simulink model "fmcw_rangemodel.slx"  (R2024b)
settings: Solver=FixedStepDiscrete  StartTime=0.0  StopTime=1.28e-3  FixedStep=5e-9  RelTol=1e-3
undefined symbols (not defined in the file or in its folder): physconst
libraries: phasedenvlib x24, phasedwavlib x6, phaseddetectlib x1
settings Model: Creator=lloyd  LastModifiedBy=lloyd

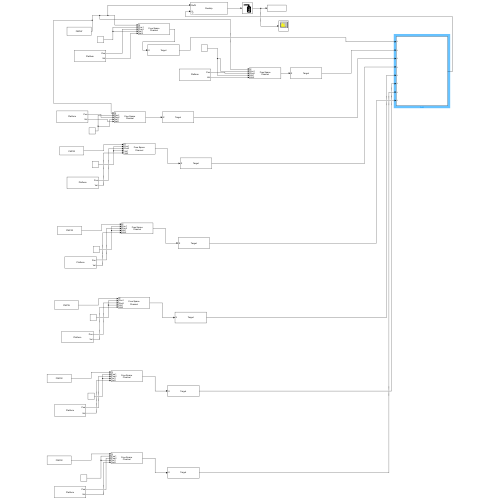
[thumbnail: Simulink's stored preview of the top-level diagram]
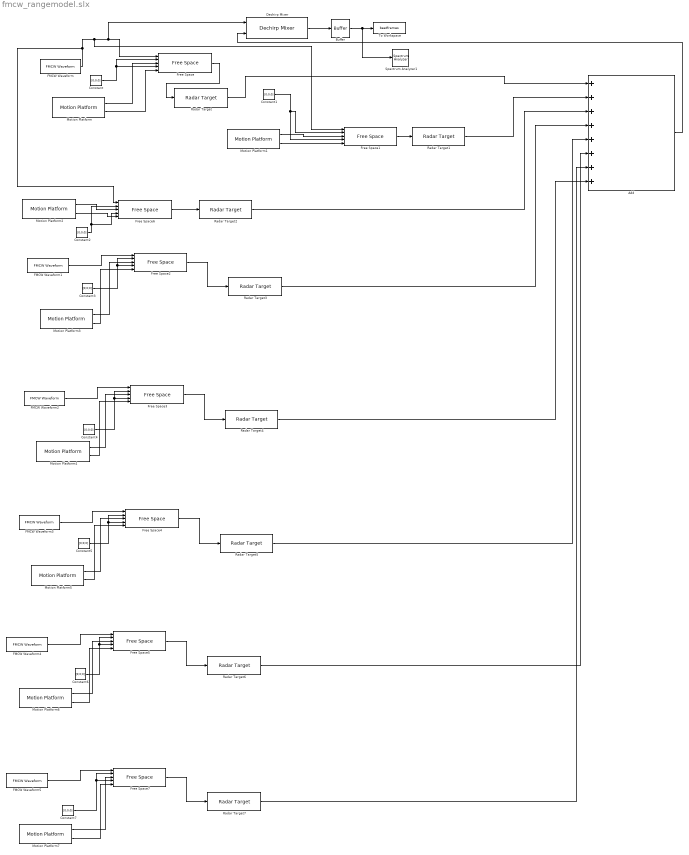
== system fmcw_rangemodel.slx ==
  Add : Sum  Inputs=++++++++
  Buffer : Buffer  N=2000  OutputFrames=off
  Constant{,1..7} (8 alike) : Constant  Value=[0;0;0]
  Dechirp Mixer : phaseddetectlib/Dechirp Mixer
  FMCW Waveform{,1..5} (6 alike) : phasedwavlib/FMCW Waveform  SampleRate=200e6  SweepTime=10e-6  SweepBandwidth=150e6  SweepDirection=Up  SweepInterval=Positive  OutputFormat=Samples  NumSamples=100  NumSweeps=1  SimulateUsing=Interpreted execution
  Free Space{,1..7} (8 alike) : phasedenvlib/Free Space  PropagationSpeed=3e8  OperatingFrequency=77e9  TwoWayPropagation=on  SampleRateFromInputCheckbox=on  SampleRate=1e6  MaximumDistanceSource=Property  MaximumDistance=500  MaximumNumInputSamplesSource=Auto  MaximumNumInputSamples=1000  SimulateUsing=Interpreted execution
  Motion Platform : phasedenvlib/Motion Platform  MotionModel=Velocity  InitialPosition=[ 50; 0; 0 ]  InitialVelocity=[ 0; 0; 0 ]  VelocitySource=Property  Velocity=[-20;0;0]  AccelerationSource=Property  Acceleration=[0;0;0]  CustomTrajectory=[ 0, 0, 0, 0, 0, 0, 0; 1, 0, 0, 0, 0, 0, 0 ]  ScanMode=None  InitialScanAngle=0  AzimuthSpan=[ -60, 60 ]  AzimuthScanRate=10  InitialOrientationAxes=eye( 3 )  OrientationAxesOutputPort=off  ElapsedTimeSource=Auto  SampleRateFromInputCheckbox=on  SampleRate=1e6  SimulateUsing=Interpreted execution
  Motion Platform1 : phasedenvlib/Motion Platform  MotionModel=Velocity  InitialPosition=[80;0;0]  InitialVelocity=[ 0; 0; 0 ]  VelocitySource=Property  Velocity=[15;0;0]  AccelerationSource=Property  Acceleration=[0;0;0]  CustomTrajectory=[ 0, 0, 0, 0, 0, 0, 0; 1, 0, 0, 0, 0, 0, 0 ]  ScanMode=None  InitialScanAngle=0  AzimuthSpan=[ -60, 60 ]  AzimuthScanRate=10  InitialOrientationAxes=eye( 3 )  OrientationAxesOutputPort=off  ElapsedTimeSource=Auto  SampleRateFromInputCheckbox=on  SampleRate=1e6  SimulateUsing=Interpreted execution
  Motion Platform2 : phasedenvlib/Motion Platform  MotionModel=Velocity  InitialPosition=[70;0;0]  InitialVelocity=[ 0; 0; 0 ]  VelocitySource=Property  Velocity=[-20;0;0]  AccelerationSource=Property  Acceleration=[0;0;0]  CustomTrajectory=[ 0, 0, 0, 0, 0, 0, 0; 1, 0, 0, 0, 0, 0, 0 ]  ScanMode=None  InitialScanAngle=0  AzimuthSpan=[ -60, 60 ]  AzimuthScanRate=10  InitialOrientationAxes=eye( 3 )  OrientationAxesOutputPort=off  ElapsedTimeSource=Auto  SampleRateFromInputCheckbox=on  SampleRate=1e6  SimulateUsing=Interpreted execution
  Motion Platform3 : phasedenvlib/Motion Platform  MotionModel=Velocity  InitialPosition=[20;0;0]  InitialVelocity=[ 0; 0; 0 ]  VelocitySource=Property  Velocity=[0;0;0]  AccelerationSource=Property  Acceleration=[0;0;0]  CustomTrajectory=[ 0, 0, 0, 0, 0, 0, 0; 1, 0, 0, 0, 0, 0, 0 ]  ScanMode=None  InitialScanAngle=0  AzimuthSpan=[ -60, 60 ]  AzimuthScanRate=10  InitialOrientationAxes=eye( 3 )  OrientationAxesOutputPort=off  ElapsedTimeSource=Auto  SampleRateFromInputCheckbox=on  SampleRate=1e6  SimulateUsing=Interpreted execution
  Motion Platform4 : phasedenvlib/Motion Platform  MotionModel=Velocity  InitialPosition=[35;0;0]  InitialVelocity=[ 0; 0; 0 ]  VelocitySource=Property  Velocity=[0;0;0]  AccelerationSource=Property  Acceleration=[0;0;0]  CustomTrajectory=[ 0, 0, 0, 0, 0, 0, 0; 1, 0, 0, 0, 0, 0, 0 ]  ScanMode=None  InitialScanAngle=0  AzimuthSpan=[ -60, 60 ]  AzimuthScanRate=10  InitialOrientationAxes=eye( 3 )  OrientationAxesOutputPort=off  ElapsedTimeSource=Auto  SampleRateFromInputCheckbox=on  SampleRate=1e6  SimulateUsing=Interpreted execution
  Motion Platform5 : phasedenvlib/Motion Platform  MotionModel=Velocity  InitialPosition=[60;0;0]  InitialVelocity=[ 0; 0; 0 ]  VelocitySource=Property  Velocity=[0;0;0]  AccelerationSource=Property  Acceleration=[0;0;0]  CustomTrajectory=[ 0, 0, 0, 0, 0, 0, 0; 1, 0, 0, 0, 0, 0, 0 ]  ScanMode=None  InitialScanAngle=0  AzimuthSpan=[ -60, 60 ]  AzimuthScanRate=10  InitialOrientationAxes=eye( 3 )  OrientationAxesOutputPort=off  ElapsedTimeSource=Auto  SampleRateFromInputCheckbox=on  SampleRate=1e6  SimulateUsing=Interpreted execution
  Motion Platform6 : phasedenvlib/Motion Platform  MotionModel=Velocity  InitialPosition=[90;0;0]  InitialVelocity=[ 0; 0; 0 ]  VelocitySource=Property  Velocity=[0;0;0]  AccelerationSource=Property  Acceleration=[0;0;0]  CustomTrajectory=[ 0, 0, 0, 0, 0, 0, 0; 1, 0, 0, 0, 0, 0, 0 ]  ScanMode=None  InitialScanAngle=0  AzimuthSpan=[ -60, 60 ]  AzimuthScanRate=10  InitialOrientationAxes=eye( 3 )  OrientationAxesOutputPort=off  ElapsedTimeSource=Auto  SampleRateFromInputCheckbox=on  SampleRate=1e6  SimulateUsing=Interpreted execution
  Motion Platform7 : phasedenvlib/Motion Platform  MotionModel=Velocity  InitialPosition=[110;0;0]  InitialVelocity=[ 0; 0; 0 ]  VelocitySource=Property  Velocity=[0;0;0]  AccelerationSource=Property  Acceleration=[0;0;0]  CustomTrajectory=[ 0, 0, 0, 0, 0, 0, 0; 1, 0, 0, 0, 0, 0, 0 ]  ScanMode=None  InitialScanAngle=0  AzimuthSpan=[ -60, 60 ]  AzimuthScanRate=10  InitialOrientationAxes=eye( 3 )  OrientationAxesOutputPort=off  ElapsedTimeSource=Auto  SampleRateFromInputCheckbox=on  SampleRate=1e6  SimulateUsing=Interpreted execution
  Radar Target : phasedenvlib/Radar Target  EnablePolarization=off  Mode=Monostatic  MeanRCSSource=Property  ScatteringMatrixSource=Property  MeanRCS=10  ScatteringMatrix=eye( 2 )  Model=Nonfluctuating  PropagationSpeed=physconst( 'LightSpeed' )  OperatingFrequency=77e9  SeedSource=Auto  Seed=0  SimulateUsing=Interpreted execution
  Radar Target1 : phasedenvlib/Radar Target  EnablePolarization=off  Mode=Monostatic  MeanRCSSource=Property  ScatteringMatrixSource=Property  MeanRCS=10  ScatteringMatrix=eye( 2 )  Model=Nonfluctuating  PropagationSpeed=physconst( 'LightSpeed' )  OperatingFrequency=77e9  SeedSource=Auto  Seed=0  SimulateUsing=Interpreted execution
  Radar Target2 : phasedenvlib/Radar Target  EnablePolarization=off  Mode=Monostatic  MeanRCSSource=Property  ScatteringMatrixSource=Property  MeanRCS=3  ScatteringMatrix=eye( 2 )  Model=Nonfluctuating  PropagationSpeed=physconst( 'LightSpeed' )  OperatingFrequency=77e9  SeedSource=Auto  Seed=0  SimulateUsing=Interpreted execution
  Radar Target{3..7} (5 alike) : phasedenvlib/Radar Target  EnablePolarization=off  Mode=Monostatic  MeanRCSSource=Property  ScatteringMatrixSource=Property  MeanRCS=1  ScatteringMatrix=eye( 2 )  Model=Nonfluctuating  PropagationSpeed=physconst( 'LightSpeed' )  OperatingFrequency=77e9  SeedSource=Auto  Seed=0  SimulateUsing=Interpreted execution
  Spectrum Analyzer1 : SpectrumAnalyzer  WindowPosition=[60.000000,203.000000,800.000000,500.000000,]  Visible=on  ScopeFrameLocation=window  WindowInvariantSamplesPerUpdate=on  Span=200000000.00000003  StartFrequency=-100000000.00000001  StopFrequency=100000000.00000001  YLimits=[-193.26599584,-98.72277309]  SelectedToolstripTab=spectrumAnalyzerToolstrip.spectrumTab
  To Workspace : ToWorkspace  VariableName=beatframes  SampleTime=-1
  wires:
  FMCW Waveform/1 -> Free Space6/1, Free Space1/1, Dechirp Mixer/1, Free Space/1
  Free Space/1 -> Radar Target/1
  Dechirp Mixer/1 -> Buffer/1
  Buffer/1 -> To Workspace/1, Spectrum Analyzer1/1
  Motion Platform/1 -> Free Space/3
  Motion Platform/2 -> Free Space/5
  Constant/1 -> Free Space/4, Free Space/2
  Motion Platform1/1 -> Free Space1/3
  Motion Platform1/2 -> Free Space1/5
  Constant1/1 -> Free Space1/4, Free Space1/2
  Free Space1/1 -> Radar Target1/1
  Radar Target/1 -> Add/1
  Radar Target1/1 -> Add/2
  Add/1 -> Dechirp Mixer/2
  FMCW Waveform1/1 -> Free Space2/1
  Free Space2/1 -> Radar Target3/1
  Free Space3/1 -> Radar Target4/1
  FMCW Waveform2/1 -> Free Space3/1
  Free Space4/1 -> Radar Target5/1
  FMCW Waveform3/1 -> Free Space4/1
  FMCW Waveform4/1 -> Free Space5/1
  Free Space5/1 -> Radar Target6/1
  Free Space6/1 -> Radar Target2/1
  Radar Target2/1 -> Add/3
  Radar Target3/1 -> Add/4
  Radar Target4/1 -> Add/8
  Radar Target5/1 -> Add/5
  Radar Target6/1 -> Add/6
  FMCW Waveform5/1 -> Free Space7/1
  Radar Target7/1 -> Add/7
  Free Space7/1 -> Radar Target7/1
  Motion Platform2/1 -> Free Space6/3
  Motion Platform2/2 -> Free Space6/5
  Constant2/1 -> Free Space6/4, Free Space6/2
  Constant3/1 -> Free Space2/4, Free Space2/2
  Motion Platform3/1 -> Free Space2/3
  Motion Platform3/2 -> Free Space2/5
  Constant4/1 -> Free Space3/4, Free Space3/2
  Motion Platform4/1 -> Free Space3/3
  Motion Platform4/2 -> Free Space3/5
  Constant5/1 -> Free Space4/4, Free Space4/2
  Motion Platform5/1 -> Free Space4/3
  Motion Platform5/2 -> Free Space4/5
  Constant6/1 -> Free Space5/4, Free Space5/2
  Motion Platform6/1 -> Free Space5/3
  Motion Platform6/2 -> Free Space5/5
  Constant7/1 -> Free Space7/4, Free Space7/2
  Motion Platform7/1 -> Free Space7/3
  Motion Platform7/2 -> Free Space7/5
